simulink model "dbsp"  (Simulink 10.1)
settings: Solver=FixedStepAuto  StartTime=0.0  StopTime=100  RelTol=1e-3
libraries: dsparch4 x2, simulink_extras x2
settings Model: Creator=iba  LastModifiedBy=iba
settings DataIOCC: SaveFormat=Dataset  SaveOutput=off  SignalLogging=off  SaveTime=off  ReturnWorkspaceOutputs=on
settings OptimizationCC: DefaultParameterBehavior=Inlined  RollThreshold=2  LifeSpan=auto
settings DebuggingCC: AlgebraicLoopMsg=error  UnderspecifiedInitializationDetection=Simplified  MergeDetectMultiDrivingBlocksExec=error  SFUnexpectedBacktrackingDiag=error  SFNoUnconditionalDefaultTransitionDiag=error  SFExecutionAtInitializationDiag=warning  ArithmeticOperatorsInVariantConditions=error
settings HardwareCC: ProdBitPerPointer=64  ProdBitPerSizeT=64  ProdBitPerPtrDiffT=64  ProdLargestAtomicFloat=Float  ProdIntDivRoundTo=Zero  ProdEndianess=LittleEndian  ProdWordSize=64  ProdHWDeviceType=Intel->x86-64 (Windows64)
settings ModelReferenceCC: PropagateSignalLabelsOutOfModel=on
settings SFSimCC: SimUseLocalCustomCode=on  CustomCodeUndefinedFunction=FilterOut
settings RTWCC: RTWUseLocalCustomCode=on
settings CodeAppCC: StateflowObjectComments=off
settings GRTTargetCC: TargetLangStandard=C99 (ISO)  CombineOutputUpdateFcns=on  GRTInterface=off
settings ConfigComp: CovMetricSettings=dwe  CovHtmlReporting=off  CovSaveCumulativeToWorkspaceVar=off  CovSaveSingleToWorkspaceVar=off  CovExternalEMLEnable=on

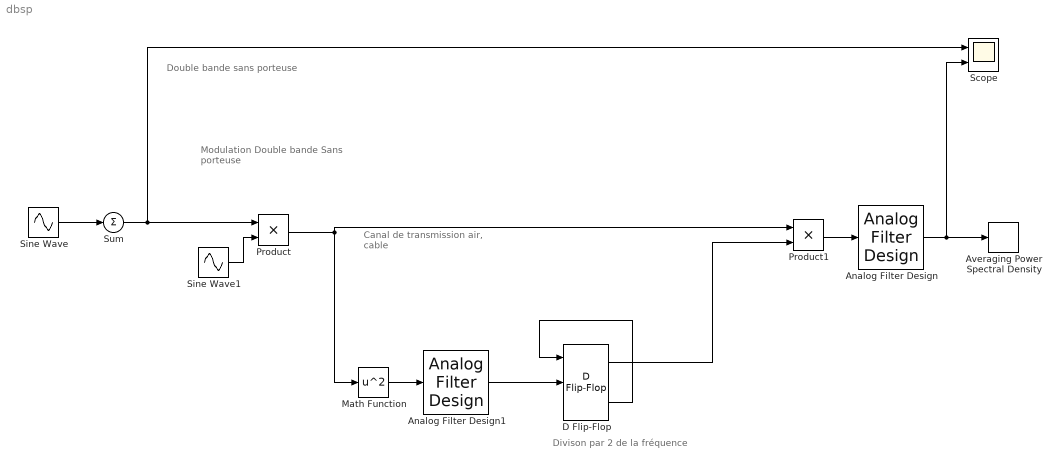
== system dbsp ==
  note: Canal de transmission
      | air, cable
  note: Modulation
      | Double bande
      | Sans porteuse
  note: Double bande sans porteuse
  note: Divison par 2
      | de la fréquence
  Analog Filter Design : dsparch4/Analog Filter Design  method=Butterworth  filttype=Lowpass  N=4  Wlo=5  Whi=80  Rp=2  Rs=40
  Analog Filter Design1 : dsparch4/Analog Filter Design  method=Chebyshev I  filttype=Bandpass  N=7  Wlo=49  Whi=51  Rp=2  Rs=40
  Averaging Power Spectral Density : simulink_extras/Additional Sinks/Averaging Power Spectral Density  npts=128*4  fftpts=512*4  HowOften=64  sampleT=0.1
      settings: SourceProductBaseCode=SL
  D Flip-Flop : simulink_extras/Flip Flops/D Flip-Flop
  Math Function : Math  Operator=square
  Product : Product
  Product1 : Product
  Scope : Scope  NumInputPorts=2
  Sine Wave : Sin  Amplitude=linspace(0.15,0.1,9)  Frequency=(1:0.5:5)  SampleTime=0.1
  Sine Wave1 : Sin  Frequency=25  SampleTime=0.1
  Sum : Sum  Inputs=+
  wires:
  Sine Wave/1 -> Sum/1
  Sum/1 -> Scope/1, Product/1
  Sine Wave1/1 -> Product/2
  Product/1 -> Product1/1, Math Function/1
  D Flip-Flop/1 -> Product1/2
  Product1/1 -> Analog Filter Design/1
  Analog Filter Design/1 -> Scope/2, Averaging Power Spectral Density/1
  Math Function/1 -> Analog Filter Design1/1
  Analog Filter Design1/1 -> D Flip-Flop/2
  D Flip-Flop/2 -> D Flip-Flop/1
